simulink model "W02_F_block_vs_hand"  (R2024b)
settings: Solver=ode4  StartTime=0  StopTime=T_final  FixedStep=h  RelTol=1e-3
values from neighbouring files (symbols this model uses):
  Kb = 2    [W02_0_setup.m]
  Kd = 4    [W02_0_setup.m]    (also in W02_E_integral.m; W02_I_tuning_by_hand.m = 1)
  Ki = 8    [W02_0_setup.m]
  Kp = 10    [W02_0_setup.m]    (also in W02_D_derivative.m; W02_E_integral.m; W02_I_tuning_by_hand.m = 5*k)
  Nf = 20    [W02_0_setup.m]    (also in W02_G_lowpass_filter.m = Nf(i))
  Nf_blk = 20    [W02_0_setup.m]
  noise_std = 0    [W02_0_setup.m]
  noise_ts = 0.01    [W02_0_setup.m]
  pid_b = 2    [W02_0_setup.m]
  pid_k = 2    [W02_0_setup.m]
  pid_m = 1    [W02_0_setup.m]
  t_step = 1    [W02_0_setup.m]
  tau_max = 1e6    (= 1000000)    [W02_0_setup.m]
  y_step = 1    [W02_0_setup.m]
libraries: slpidlib x1
settings Model: Creator=admin  LastModifiedBy=admin
settings DataIOCC: ReturnWorkspaceOutputs=off

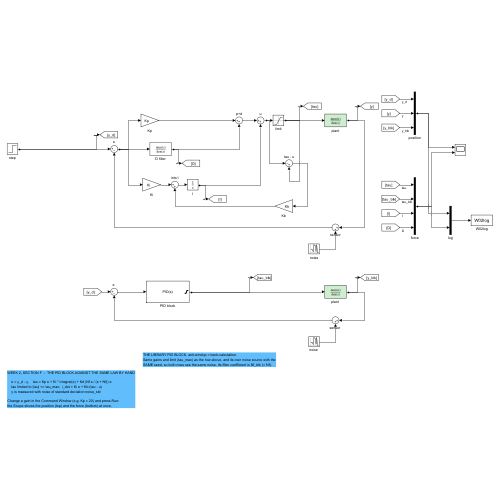
[thumbnail: Simulink's stored preview of the top-level diagram]
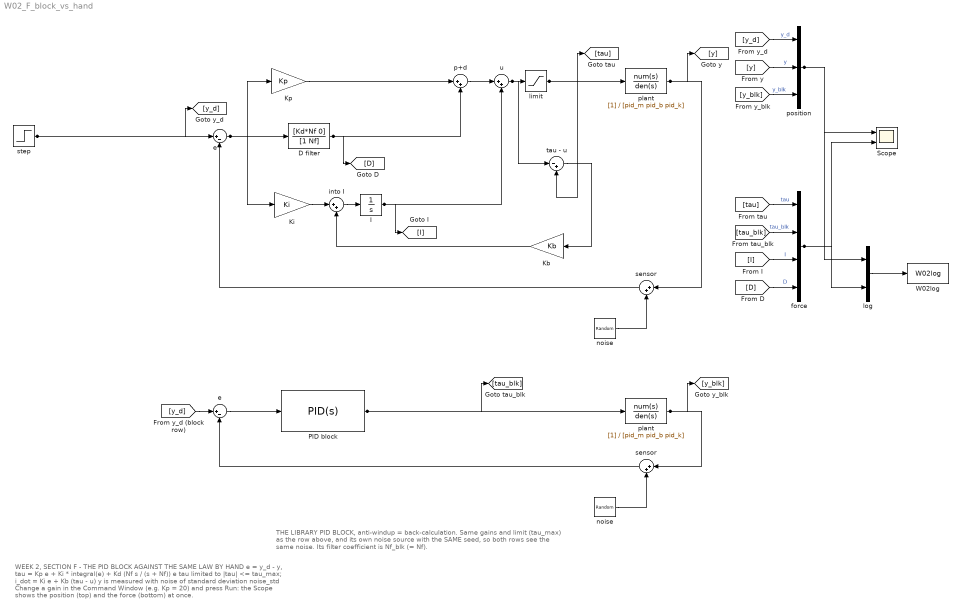
== system W02_F_block_vs_hand ==
  note: THE LIBRARY PID BLOCK, anti-windup = back-calculation.
      | Same gains and limit (tau_max) as the row above, and its own noise source with the
      | SAME seed, so both rows see the same noise. Its filter coefficient is Nf_blk (= Nf).
  note: WEEK 2, SECTION F  -  THE PID BLOCK AGAINST THE SAME LAW BY HAND
      |
      |     e = y_d - y,    tau = Kp e + Ki * integral(e) + Kd (Nf s / (s + Nf)) e
      |     tau limited to |tau| <= tau_max;  i_dot = Ki e + Kb (tau - u)
      |     y is measured with noise of standard deviation noise_std
      |
      | Change a gain in the Command Window (e.g. Kp = 20) and press Run:
      | the Scope shows the position (top) and the force (bottom) at once.
  D filter : TransferFcn  Numerator=[Kd*Nf 0]  Denominator=[1 Nf]
  I : Integrator
  Kb : Gain  Gain=Kb
  Ki : Gain  Gain=Ki
  Kp : Gain  Gain=Kp
  PID block : slpidlib/PID Controller  Controller=PID  Form=Parallel  TimeDomain=Continuous-time  UseExternalTs=off  SampleTime=-1  IntegratorMethod=Forward Euler  FilterMethod=Forward Euler  ControllerParametersSource=internal  P=Kp  I=Ki  UseKiTs=off  D=Kd  UseExternalDerivativeSource=off  N=Nf_blk  UseFilter=on  TunerSelectOption=Transfer Function Based (PID Tuner App)  InitialConditionSource=internal  InitialConditionForIntegrator=0  InitialConditionForFilter=0  DifferentiatorICPrevScaledInput=0  ExternalReset=none  TrackingMode=off  Kt=1  LimitOutput=on  SatLimitsSource=internal  UpperSaturationLimit=tau_max  LowerSaturationLimit=-tau_max  LinearizeAsGain=on  AntiWindupMode=back-calculation  Kb=Kb  LimitIntegrator=off  UpperIntegratorSaturationLimit=inf  LowerIntegratorSaturationLimit=-inf  POutMin=[]  POutMax=[]  IOutMin=[]  IOutMax=[]  DOutMin=[]  DOutMax=[]  NOutMin=[]  NOutMax=[]  SumOutMin=[]  SumOutMax=[]  SaturationOutMin=[]  SaturationOutMax=[]  PParamMin=[]  PParamMax=[]  IParamMin=[]  IParamMax=[]  DParamMin=[]  DParamMax=[]  NParamMin=[]  NParamMax=[]  KbParamMin=[]  KbParamMax=[]  KtParamMin=[]  KtParamMax=[]  KbOutMin=[]  KbOutMax=[]  KtOutMin=[]  KtOutMax=[]  IntegratorOutMin=[]  IntegratorOutMax=[]  FilterOutMin=[]  FilterOutMax=[]  SumI1OutMin=[]  SumI1OutMax=[]  SumI2OutMin=[]  SumI2OutMax=[]  SumI3OutMin=[]  SumI3OutMax=[]  SumI4OutMin=[]  SumI4OutMax=[]  SumDOutMin=[]  SumDOutMax=[]  DifferentiatorOutMin=[]  DifferentiatorOutMax=[]  FilterDiffOutCoefMin=[]  FilterDiffOutCoefMax=[]  ReciprocalOutMin=[]  ReciprocalOutMax=[]  SumDenOutMin=[]  SumDenOutMax=[]  SumNumOutMin=[]  SumNumOutMax=[]  DivideOutMin=[]  DivideOutMax=[]  UdiffTsProdOutMin=[]  UdiffTsProdOutMax=[]  NTsProdOutMin=[]  NTsProdOutMax=[]  UintegralTsProdOutMin=[]  UintegralTsProdOutMax=[]  UngainTsProdOutMin=[]  UngainTsProdOutMax=[]  ClampingZeroOutDataTypeStr=Inherit: Inherit via back propagation  ClampingZeroOutMin=[]  ClampingZeroOutMax=[]  FilterDenConstantOutDataTypeStr=Inherit: Inherit via back propagation  FilterDenConstantOutMin=[]  FilterDenConstantOutMax=[]  PCopyOutDataTypeStr=Inherit: Inherit via back propagation  PCopyOutMin=[]  PCopyOutMax=[]  NCopyOutDataTypeStr=Inherit: Inherit via back propagation  NCopyOutMin=[]  NCopyOutMax=[]  IntegratorContinuousStateAttributes=''  IntegratorStateMustResolveToSignalObject=off  IntegratorRTWStateStorageClass=Auto  FilterContinuousStateAttributes=''  FilterStateMustResolveToSignalObject=off  FilterRTWStateStorageClass=Auto  ParallelPVariant=InternalParameters  IdealPVariant=Disabled  IVariant=InternalParameters  DVariant=InternalParameters  IntegratorVariant=Continuous  SatVariant=Enabled  AWVariant=BackCalculation  PCopyVariant=Disabled  TRVariant=Disabled  FdbkBlocksVariant=Forward  IdealPFdbkVariant=Disabled  SatFdbkVariant=Disabled  DerivativeFilterVariant=ContFilter  NVariant=InternalParameters  NCopyVariant=Disabled  FilterICVariant=InternalICsFilter  IntegratorICVariant=InternalICs  ExternalResetVariant=Disabled  TRSumVariant=Passthrough  SumFdbkVariant=Disabled  SumVariant=Sum_PID  TsampFilterVariant=InternalTs  TsampNgainVariant=Passthrough  TsampIntegralVariant=Disabled_SignalSpec  ExternalSaturationOutDataTypeStr=Inherit: Same as second input  DerivativeSourceVariant=ErrorSignal  PreIntVariant=InternalPreInt
  Scope : Scope  NumInputPorts=2
  W02log : ToWorkspace  VariableName=W02log  SaveFormat=Structure With Time  SampleTime=-1
  e : Sum  Inputs=|+-
  "e " : Sum  Inputs=|+-
  force : Mux
  into I : Sum  Inputs=|++
  limit : Saturate  UpperLimit=tau_max  LowerLimit=-tau_max
  log : Mux  Inputs=2
  noise : RandomNumber  Variance=noise_std^2  Seed=23341  SampleTime=noise_ts
  "noise " : RandomNumber  Variance=noise_std^2  Seed=23341  SampleTime=noise_ts
  p+d : Sum  Inputs=|++
  plant : TransferFcn  Denominator=[pid_m pid_b pid_k]
  "plant " : TransferFcn  Denominator=[pid_m pid_b pid_k]
  position : Mux  Inputs=3
  sensor : Sum  Inputs=|++
  "sensor " : Sum  Inputs=|++
  step : Step  Time=t_step  After=y_step  SampleTime=0
  tau - u : Sum  Inputs=|-+
  u : Sum  Inputs=|++
  wires:
  step/1 -> e/1, [y_d]
  e/1 -> Kp/1, D filter/1, Ki/1
  Kp/1 -> p+d/1
  D filter/1 -> p+d/2, [D]
  Ki/1 -> into I/1
  into I/1 -> I/1
  p+d/1 -> u/1
  I/1 -> u/2, [I]
  u/1 -> limit/1, tau - u/1
  limit/1 -> tau - u/2, plant/1, [tau]
  tau - u/1 -> Kb/1
  Kb/1 -> into I/2
  plant/1 -> [y], sensor/1
  noise/1 -> sensor/2
  sensor/1 -> e/2
  [y_d] -> "e "/1
  "e "/1 -> PID block/1
  PID block/1 -> "plant "/1, [tau_blk]
  "plant "/1 -> [y_blk], "sensor "/1
  "noise "/1 -> "sensor "/2
  "sensor "/1 -> "e "/2
  [y_d] -> position/1  "y_d"
  [y] -> position/2  "y"
  [y_blk] -> position/3  "y_blk"
  [tau] -> force/1  "tau"
  [tau_blk] -> force/2  "tau_blk"
  [I] -> force/3  "I"
  [D] -> force/4  "D"
  position/1 -> Scope/1, log/1
  force/1 -> Scope/2, log/2
  log/1 -> W02log/1
